simulink model "VSI"  (Simulink 8.2)
settings: Solver=ode23t  StartTime=0  StopTime=0.01  MaxStep=.1e-6  RelTol=1e-4  AbsTol=1e-5
values from neighbouring files (symbols this model uses):
  Ca = 1/1*32e-6    (= 3.2e-05)    [VSI_AFE_parameters_LC_900Hz.m]    (also in VSI_AFE_parameters_LC_9kHz.m = 1.6e-05)
  Cc = 1/1*31.8e-6    (= 3.18e-05)    [VSI_AFE_parameters_LC_900Hz.m]    (also in VSI_AFE_parameters_LC_9kHz.m = 1.59e-05)
  Cdc_vsi = 147.3e-6    (= 0.0001473)    [VSI_AFE_parameters_LC_900Hz.m]    (also in VSI_AFE_parameters_LC_9kHz.m)
  DeadTime = 0*0.5e-6    (= 0)    [VSI_AFE_parameters_LC_900Hz.m]    (also in VSI_AFE_parameters_LC_9kHz.m)
  FWPI_a1 = 0.08921    [VSI_AFE_parameters_LC_900Hz.m]    (also in VSI_AFE_parameters_LC_9kHz.m)
  FWPI_a2 = -0.08901    [VSI_AFE_parameters_LC_900Hz.m]    (also in VSI_AFE_parameters_LC_9kHz.m)
  Kii_AFE = 46.5421*270    (= 12566.367)    [VSI_AFE_parameters_LC_900Hz.m]    (also in VSI_AFE_parameters_LC_9kHz.m)
  Kii_VSI = 121.0095*270    (= 32672.565)    [VSI_AFE_parameters_LC_900Hz.m]    (also in VSI_AFE_parameters_LC_9kHz.m)
  Kiv_AFE = 4.5815    [VSI_AFE_parameters_LC_900Hz.m]    (also in VSI_AFE_parameters_LC_9kHz.m)
  Kiv_VSI = 130.8997    [VSI_AFE_parameters_LC_900Hz.m]    (also in VSI_AFE_parameters_LC_9kHz.m)
  Kpi_AFE = 0.0116*270    (= 3.132)    [VSI_AFE_parameters_LC_900Hz.m]    (also in VSI_AFE_parameters_LC_9kHz.m)
  Kpi_VSI = 0.0465*270    (= 12.555)    [VSI_AFE_parameters_LC_900Hz.m]    (also in VSI_AFE_parameters_LC_9kHz.m)
  Kpv_AFE = 0.0462    [VSI_AFE_parameters_LC_900Hz.m]    (also in VSI_AFE_parameters_LC_9kHz.m)
  Kpv_VSI = 0.0495    [VSI_AFE_parameters_LC_900Hz.m]    (also in VSI_AFE_parameters_LC_9kHz.m)
  La = 1/1*962e-6    (= 0.000962)    [VSI_AFE_parameters_LC_900Hz.m]    (also in VSI_AFE_parameters_LC_9kHz.m = 1.924e-05)
  Lb = 1/1*985e-6    (= 0.000985)    [VSI_AFE_parameters_LC_900Hz.m]    (also in VSI_AFE_parameters_LC_9kHz.m = 1.97e-05)
  Lc = 1/1*972e-6    (= 0.000972)    [VSI_AFE_parameters_LC_900Hz.m]    (also in VSI_AFE_parameters_LC_9kHz.m = 1.944e-05)
  LCa = 0.61e-6    (= 6.1e-07)    [VSI_AFE_parameters_LC_900Hz.m]    (also in VSI_AFE_parameters_LC_9kHz.m)
  LCb = 0.61e-6    (= 6.1e-07)    [VSI_AFE_parameters_LC_900Hz.m]    (also in VSI_AFE_parameters_LC_9kHz.m)
  LCc = 0.63e-6    (= 6.3e-07)    [VSI_AFE_parameters_LC_900Hz.m]    (also in VSI_AFE_parameters_LC_9kHz.m)
  LCdc_vsi = 0.57e-6    (= 5.7e-07)    [VSI_AFE_parameters_LC_900Hz.m]    (also in VSI_AFE_parameters_LC_9kHz.m)
  PWM_Cycle = 4000    [VSI_AFE_parameters_LC_900Hz.m]    (also in VSI_AFE_parameters_LC_9kHz.m)
  R = 12    [VSI_AFE_parameters_LC_900Hz.m]    (also in VSI_AFE_parameters_LC_9kHz.m)
  RCa = 0.051    [VSI_AFE_parameters_LC_900Hz.m]    (also in VSI_AFE_parameters_LC_9kHz.m)
  RCb = 0.054    [VSI_AFE_parameters_LC_900Hz.m]    (also in VSI_AFE_parameters_LC_9kHz.m)
  RCc = 0.052    [VSI_AFE_parameters_LC_900Hz.m]    (also in VSI_AFE_parameters_LC_9kHz.m)
  RCdc_vsi = 0.046    [VSI_AFE_parameters_LC_900Hz.m]    (also in VSI_AFE_parameters_LC_9kHz.m)
  RLa = 0.123    [VSI_AFE_parameters_LC_900Hz.m]    (also in VSI_AFE_parameters_LC_9kHz.m)
  RLb = 0.132    [VSI_AFE_parameters_LC_900Hz.m]    (also in VSI_AFE_parameters_LC_9kHz.m)
  RLc = 0.089    [VSI_AFE_parameters_LC_900Hz.m]    (also in VSI_AFE_parameters_LC_9kHz.m)
  Vdc = 270/1    (= 270)    [VSI_AFE_parameters_LC_900Hz.m]    (also in VSI_AFE_parameters_LC_9kHz.m)
undefined symbols (not defined in the file or in its folder): Cdc, Ldc
libraries: powerlib x27, cstblocks x10, powerlib_extras x3, simulink x2
settings Model: Creator=marko  LastModifiedBy=wenbo
settings SolverCC: MaxConsecutiveMinStep=10  ZeroCrossAlgorithm=Adaptive  AlgebraicLoopSolver=LineSearch
settings DataIOCC: LimitDataPoints=off  SaveFinalState=on
settings DebuggingCC: IgnoredZcDiagnostic=none  FcnCallInpInsideContextMsg=EnableAllAsWarning

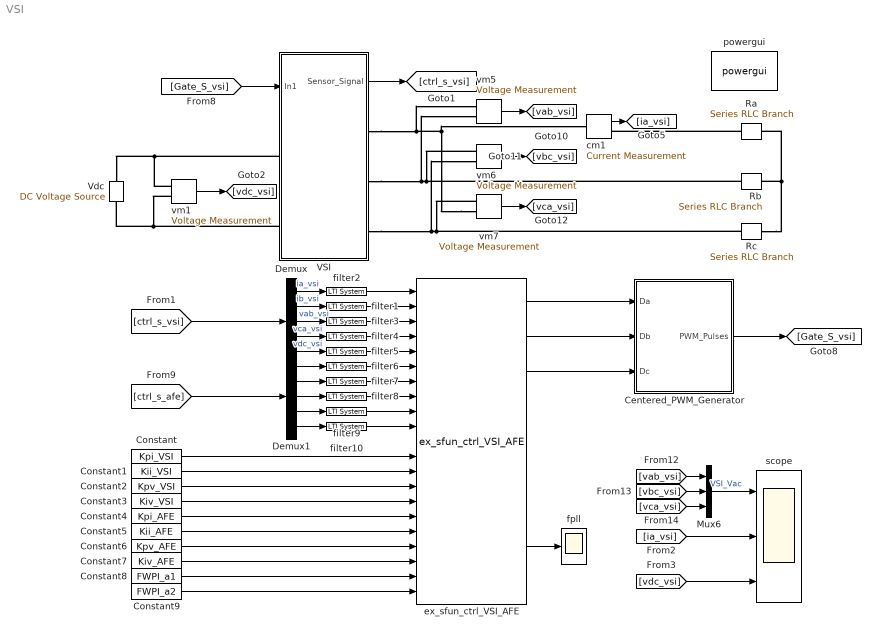
== system VSI ==
  Centered_PWM_Generator : Subsystem
  Constant : Constant  Value=Kpi_VSI
  Constant1 : Constant  Value=Kii_VSI
  Constant2 : Constant  Value=Kpv_VSI
  Constant3 : Constant  Value=Kiv_VSI
  Constant4 : Constant  Value=Kpi_AFE
  Constant5 : Constant  Value=Kii_AFE
  Constant6 : Constant  Value=Kpv_AFE
  Constant7 : Constant  Value=Kiv_AFE
  Constant8 : Constant  Value=FWPI_a1
  Constant9 : Constant  Value=FWPI_a2
  Demux : Demux  Outputs=5
  Demux1 : Demux  Outputs=5
  Mux6 : Mux  Inputs=3
  Ra : powerlib/Elements/Series RLC Branch  LConnTagsString=__new0  RConnTagsString=__new0  BranchType=R  Resistance=R  Inductance=Ldc  SetiL0=off  InitialCurrent=0  Capacitance=Cdc  Setx0=off  InitialVoltage=0  Measurements=None
  Rb : powerlib/Elements/Series RLC Branch  LConnTagsString=__new0  RConnTagsString=__new0  BranchType=R  Resistance=R  Inductance=Ldc  SetiL0=off  InitialCurrent=0  Capacitance=Cdc  Setx0=off  InitialVoltage=0  Measurements=None
  Rc : powerlib/Elements/Series RLC Branch  LConnTagsString=__new0  RConnTagsString=__new0  BranchType=R  Resistance=R  Inductance=Ldc  SetiL0=off  InitialCurrent=0  Capacitance=Cdc  Setx0=off  InitialVoltage=0  Measurements=None
  VSI : Subsystem
  Vdc : powerlib/Electrical Sources/DC Voltage Source  Amplitude=Vdc  Measurements=None
  cm1 : powerlib/Measurements/Current Measurement  PhasorSimulation=off  OutputType=Complex  PSBequivalent=0
  ex_sfun_ctrl_VSI_AFE : S-Function  FunctionName=ex_sfun_ctrl_VSI_AFE  EnableBusSupport=off
  filter{1..10} (10 alike) : cstblocks/LTI System  sys=tf_filter  IC=[]
  fpll : Scope
      settings: TimeRange=0.4  YMin=-150  YMax=60  SaveName=ia_L1
  powergui : powerlib/powergui  Priority=1  SimulationMode=Continuous  SolverType=Tustin  SampleTime=50e-6  frequency=60  SPID=on  DisableSnubberDevices=off  DisableRonSwitches=off  DisableVfSwitches=off  SwTol=0  Interpol=off  DisplayEquations=off  frequencyindice=0  Pbase=100e6  ErrMax=1e-4  Iterations=50  UnitsV=kV  UnitsW=MW  FunctionMessages=off  echomessages=off  HookPort=off  EnableUseOfTLC=off  x0status=blocks  RestoreLinks=warning  ResistiveCurrentMeasurement=off  Frange=[0:2:500]  Ylog=off  Xlog=on  ShowGrid=off  save=off  variable=ZData  structure=ia_L  ZoomFFT=on  StartTime=0.1  cycles=1  DisplayStyle=1  fundamental=400  FreqAxis=off  MaxFrequency=100000  frequencyindicesteady=400  RmsSteady=1  display=off  Ts=0  methode=off
  scope : Scope  NumInputPorts=3
      settings: YMin=-150~-8~-1  YMax=150~8~1  SaveName=va_ia  MaxDataPoints=2000000
  vm{1,5..7} (4 alike) : powerlib/Measurements/Voltage Measurement  PhasorSimulation=off  OutputType=Complex  PSBequivalent=0
  wires:
  vm5/1 -> [vab_vsi]
  vm6/1 -> [vbc_vsi]
  vm7/1 -> [vca_vsi]
  [vab_vsi] -> Mux6/1
  [vbc_vsi] -> Mux6/2
  [vca_vsi] -> Mux6/3
  Mux6/1 -> scope/1  "VSI_Vac"
  Centered_PWM_Generator/1(PWM_Pulses) -> [Gate_S_vsi]
  VSI/1(Sensor_Signal) -> [ctrl_s_vsi]
  [Gate_S_vsi] -> VSI/1(In1)
  [ctrl_s_afe] -> Demux1/1
  ex_sfun_ctrl_VSI_AFE/1 -> Centered_PWM_Generator/1(Da)
  ex_sfun_ctrl_VSI_AFE/2 -> Centered_PWM_Generator/2(Db)
  ex_sfun_ctrl_VSI_AFE/3 -> Centered_PWM_Generator/3(Dc)
  ex_sfun_ctrl_VSI_AFE/8 -> fpll/1
  cm1/1 -> [ia_vsi]
  [ia_vsi] -> scope/2
  [vdc_vsi] -> scope/3
  [ctrl_s_vsi] -> Demux/1
  Demux/1 -> filter2/1  "ia_vsi"
  Demux/2 -> filter1/1  "ib_vsi"
  Demux/3 -> filter3/1  "vab_vsi"
  Demux/4 -> filter4/1  "vca_vsi"
  Demux/5 -> filter5/1  "vdc_vsi"
  Demux1/1 -> filter6/1
  Demux1/2 -> filter7/1
  Demux1/3 -> filter8/1
  Demux1/4 -> filter9/1
  Demux1/5 -> filter10/1
  Constant/1 -> ex_sfun_ctrl_VSI_AFE/12
  Constant1/1 -> ex_sfun_ctrl_VSI_AFE/13
  Constant2/1 -> ex_sfun_ctrl_VSI_AFE/14
  Constant3/1 -> ex_sfun_ctrl_VSI_AFE/15
  Constant4/1 -> ex_sfun_ctrl_VSI_AFE/16
  Constant5/1 -> ex_sfun_ctrl_VSI_AFE/17
  Constant6/1 -> ex_sfun_ctrl_VSI_AFE/18
  Constant7/1 -> ex_sfun_ctrl_VSI_AFE/19
  Constant8/1 -> ex_sfun_ctrl_VSI_AFE/20
  Constant9/1 -> ex_sfun_ctrl_VSI_AFE/21
  filter2/1 -> ex_sfun_ctrl_VSI_AFE/1
  filter1/1 -> ex_sfun_ctrl_VSI_AFE/2
  filter3/1 -> ex_sfun_ctrl_VSI_AFE/3
  filter4/1 -> ex_sfun_ctrl_VSI_AFE/4
  filter5/1 -> ex_sfun_ctrl_VSI_AFE/5
  filter6/1 -> ex_sfun_ctrl_VSI_AFE/6
  filter7/1 -> ex_sfun_ctrl_VSI_AFE/7
  filter8/1 -> ex_sfun_ctrl_VSI_AFE/8
  filter9/1 -> ex_sfun_ctrl_VSI_AFE/9
  filter10/1 -> ex_sfun_ctrl_VSI_AFE/10
  vm1/1 -> [vdc_vsi]
  connections:
  VSI/LConn1 -- vm1/LConn1 -- Vdc/RConn1
  VSI/LConn2 -- vm1/LConn2 -- Vdc/LConn1
  vm7/LConn1 -- VSI/RConn3 -- vm6/LConn2 -- Rc/RConn1
  vm6/LConn1 -- VSI/RConn2 -- vm5/LConn2 -- Rb/RConn1
  Rb/LConn1 -- Rc/LConn1 -- Ra/LConn1
  vm7/LConn2 -- VSI/RConn1 -- vm5/LConn1 -- cm1/LConn1
  Ra/RConn1 -- cm1/RConn1

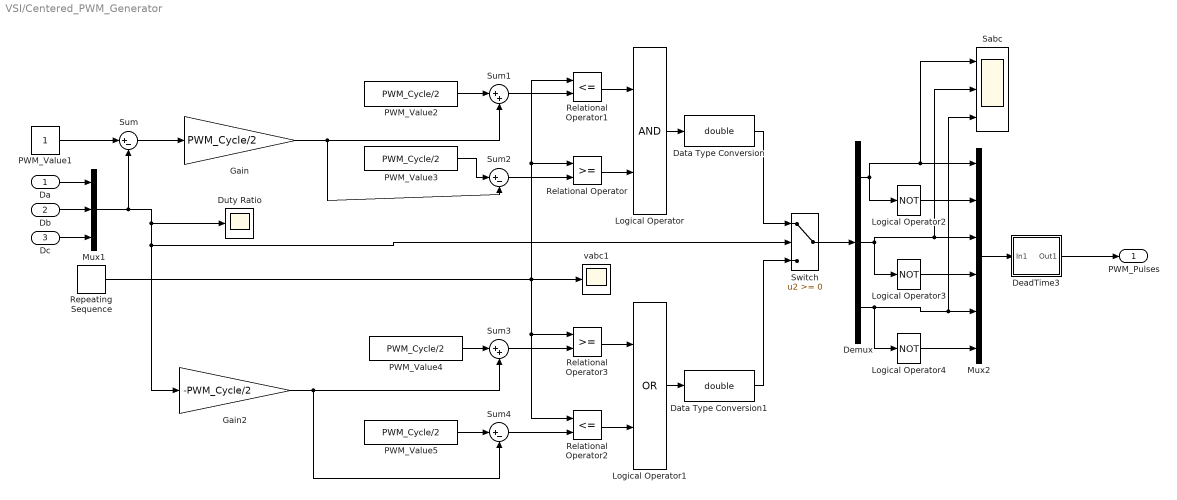
== system VSI/Centered_PWM_Generator ==
  Da : Inport
  Db : Inport  Port=2
  Dc : Inport  Port=3
  Data Type Conversion : DataTypeConversion  OutDataTypeStr=double
  Data Type Conversion1 : DataTypeConversion  OutDataTypeStr=double
  DeadTime3 : Subsystem
  Demux : Demux  Outputs=3
  Duty Ratio : Scope
      settings: TimeRange=0.01  YMin=0.25  YMax=0.75  SaveName=vabcll1
  Gain : Gain  Gain=PWM_Cycle/2
  Gain2 : Gain  Gain=-PWM_Cycle/2
  Logical Operator : Logic  AllPortsSameDT=off  OutDataTypeStr=boolean
  Logical Operator1 : Logic  Operator=OR  AllPortsSameDT=off  OutDataTypeStr=boolean
  Logical Operator2 : Logic  Operator=NOT  OutDataTypeStr=float('double')
  Logical Operator3 : Logic  Operator=NOT  OutDataTypeStr=float('double')
  Logical Operator4 : Logic  Operator=NOT  OutDataTypeStr=float('double')
  Mux1 : Mux  Inputs=3
  Mux2 : Mux  Inputs=6
  PWM_Value1 : Constant
  PWM_Value{2..5} (4 alike) : Constant  Value=PWM_Cycle/2
  Relational Operator : RelationalOperator  OutDataTypeStr=boolean
  Relational Operator1 : RelationalOperator  Operator=<=  OutDataTypeStr=boolean
  Relational Operator2 : RelationalOperator  Operator=<=  OutDataTypeStr=boolean
  Relational Operator3 : RelationalOperator  OutDataTypeStr=boolean
  Repeating Sequence : simulink/Sources/Repeating Sequence  rep_seq_t="[0  (PWM_Cycle*12.5e-9)]"  rep_seq_y=[0 PWM_Cycle]
  Sabc : Scope  NumInputPorts=3
      settings: TimeRange=0.0005  YMin=-9~-5~-5  YMax=8~5~5  SaveName=iabc_L2
  Sum : Sum  Inputs=|+-
  Sum1 : Sum  Inputs=|++
  Sum2 : Sum  Inputs=|+-
  Sum3 : Sum  Inputs=|++
  Sum4 : Sum  Inputs=|+-
  Switch : Switch
  vabc1 : Scope
      settings: TimeRange=0.01  YMin=0  YMax=4000  SaveName=vabcll2
  PWM_Pulses : Outport
  wires:
  Logical Operator4/1 -> Mux2/6
  Demux/3 -> Logical Operator4/1, Mux2/5, Sabc/3
  Logical Operator3/1 -> Mux2/4
  Demux/2 -> Mux2/3, Sabc/2, Logical Operator3/1
  Logical Operator2/1 -> Mux2/2
  Demux/1 -> Mux2/1, Sabc/1, Logical Operator2/1
  Mux2/1 -> DeadTime3/1(In1)
  Dc/1 -> Mux1/3
  Db/1 -> Mux1/2
  Da/1 -> Mux1/1
  Mux1/1 -> Sum/2, Gain2/1, Switch/2, Duty Ratio/1
  Switch/1 -> Demux/1
  Data Type Conversion1/1 -> Switch/3
  Gain2/1 -> Sum3/2, Sum4/2
  Logical Operator1/1 -> Data Type Conversion1/1
  Relational Operator2/1 -> Logical Operator1/2
  Relational Operator3/1 -> Logical Operator1/1
  Sum3/1 -> Relational Operator3/2
  Sum4/1 -> Relational Operator2/2
  PWM_Value5/1 -> Sum4/1
  PWM_Value4/1 -> Sum3/1
  Data Type Conversion/1 -> Switch/1
  Logical Operator/1 -> Data Type Conversion/1
  Relational Operator/1 -> Logical Operator/2
  Relational Operator1/1 -> Logical Operator/1
  Sum1/1 -> Relational Operator1/2
  Sum2/1 -> Relational Operator/2
  PWM_Value3/1 -> Sum2/1
  Gain/1 -> Sum2/2, Sum1/2
  Sum/1 -> Gain/1
  PWM_Value1/1 -> Sum/1
  Repeating Sequence/1 -> vabc1/1, Relational Operator1/1, Relational Operator/1, Relational Operator3/1, Relational Operator2/1
  DeadTime3/1(Out1) -> PWM_Pulses/1
  PWM_Value2/1 -> Sum1/1

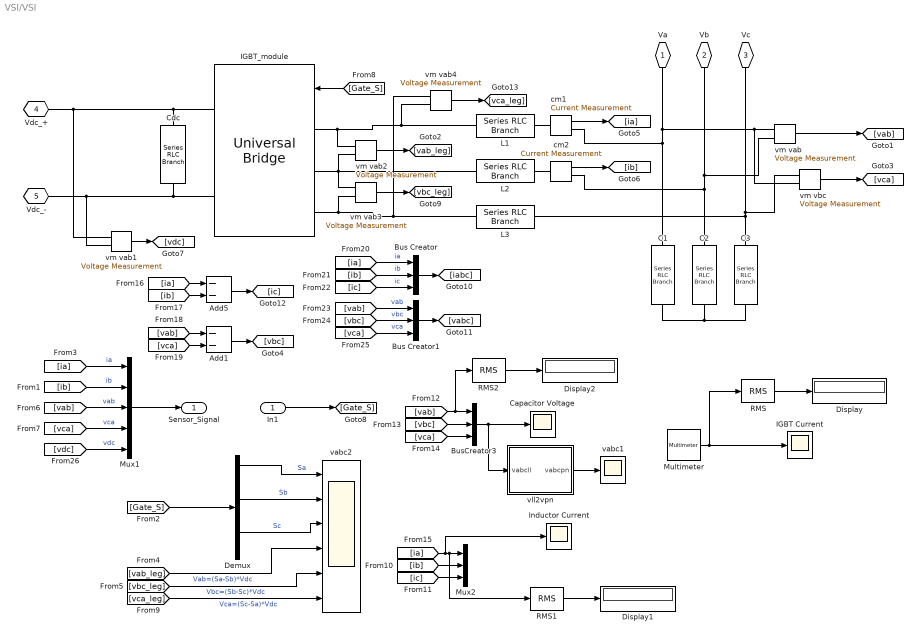
== system VSI/VSI ==
  In1 : Inport
  Add1 : Sum  Inputs=--
  Add5 : Sum  Inputs=--
  Bus Creator : BusCreator  Inputs=3
  Bus Creator1 : BusCreator  Inputs=3
  BusCreator3 : BusCreator  Inputs=3
  C1 : powerlib/Elements/Series RLC Branch  LConnTagsString=__new0  RConnTagsString=__new0  BranchType=RC  Resistance=RCa  Inductance=LCa  SetiL0=off  InitialCurrent=0  Capacitance=Ca  Setx0=off  InitialVoltage=0  Measurements=None
  C2 : powerlib/Elements/Series RLC Branch  LConnTagsString=__new0  RConnTagsString=__new0  BranchType=RC  Resistance=RCb  Inductance=LCb  SetiL0=off  InitialCurrent=0  Capacitance=Cc  Setx0=off  InitialVoltage=0  Measurements=None
  C3 : powerlib/Elements/Series RLC Branch  LConnTagsString=__new0  RConnTagsString=__new0  BranchType=RC  Resistance=RCc  Inductance=LCc  SetiL0=off  InitialCurrent=0  Capacitance=Cc  Setx0=off  InitialVoltage=0  Measurements=None
  Capacitor Voltage : Scope
      settings: TimeRange=0.06  YMin=-300  YMax=225  SaveName=vabcll
  Cdc : powerlib/Elements/Series RLC Branch  LConnTagsString=__new0  RConnTagsString=__new0  BranchType=RC  Resistance=RCdc_vsi  Inductance=LCdc_vsi  SetiL0=off  InitialCurrent=0  Capacitance=Cdc_vsi  Setx0=off  InitialVoltage=0  Measurements=None
  Demux : Demux  Outputs=6
  Display : Display
  Display1 : Display
  Display2 : Display
  IGBT Current : Scope
      settings: TimeRange=0.01  YMin=-80  YMax=80  SaveName=I_IGBT
  IGBT_module : powerlib/Power Electronics/Universal Bridge  Arms=3  SnubberResistance=inf  SnubberCapacitance=inf  Device=IGBT / Diodes  Ron=0  Lon=0  ForwardVoltages=[0 0]  ForwardVoltage=0  GTOparameters=[ 10e-6 , 20e-6 ]  IGBTparameters=[ 0, 0 ]  Measurements=All voltages and currents  Measurements_2=None  converterType=Rectifier
  Inductor Current : Scope
      settings: TimeRange=0.06  YMin=-35  YMax=35  SaveName=Ia_L
  L1 : powerlib/Elements/Series RLC Branch  LConnTagsString=__new0  RConnTagsString=__new0  BranchType=RL  Resistance=RLa  Inductance=La  SetiL0=off  InitialCurrent=0  Capacitance=1e-6  Setx0=off  InitialVoltage=0  Measurements=None
  L2 : powerlib/Elements/Series RLC Branch  LConnTagsString=__new0  RConnTagsString=__new0  BranchType=RL  Resistance=RLb  Inductance=Lb  SetiL0=off  InitialCurrent=0  Capacitance=1e-6  Setx0=off  InitialVoltage=0  Measurements=None
  L3 : powerlib/Elements/Series RLC Branch  LConnTagsString=__new0  RConnTagsString=__new0  BranchType=RL  Resistance=RLc  Inductance=Lc  SetiL0=off  InitialCurrent=0  Capacitance=1e-6  Setx0=off  InitialVoltage=0  Measurements=None
  Multimeter : powerlib/Measurements/Multimeter  PhasorSimulation=off  OutputType=Complex  sel=11  L=16  Gain=1  yselected={'Isw1: VSI/IGBT_module'};  PSBOutputType=1  PSBequivalent=0  AxesSetting=[0,0.1,-100,100]  Display=0  SavedBlockNames=-11
  Mux1 : Mux  Inputs=5
  Mux2 : Mux  Inputs=3
  RMS : powerlib_extras/Measurements/RMS  f1=400
  RMS1 : powerlib_extras/Measurements/RMS  f1=400
  RMS2 : powerlib_extras/Measurements/RMS  f1=400
  cm1 : powerlib/Measurements/Current Measurement  PhasorSimulation=off  OutputType=Complex  PSBequivalent=0
  cm2 : powerlib/Measurements/Current Measurement  PhasorSimulation=off  OutputType=Complex  PSBequivalent=0
  vabc1 : Scope
      settings: TimeRange=0.01  YMin=-80  YMax=80  SaveName=vabc
  vabc2 : Scope  NumInputPorts=6
      settings: YMin=0~0~0~-300~-300~-300  YMax=1~1~1~300~300~300  SaveName=gate_vab
  vll2vpn : Subsystem
  vm vab{,1..4} (5 alike) : powerlib/Measurements/Voltage Measurement  PhasorSimulation=off  OutputType=Complex  PSBequivalent=0
  vm vbc : powerlib/Measurements/Voltage Measurement  PhasorSimulation=off  OutputType=Complex  PSBequivalent=0
  Va : PMIOPort  Tag=PMCPort  Port=1  Side=Right
  Vb : PMIOPort  Tag=PMCPort  Port=2  Side=Right
  Vc : PMIOPort  Tag=PMCPort  Port=3  Side=Right
  Vdc_+ : PMIOPort  Tag=PMCPort  Port=4  Side=Left
  Vdc_- : PMIOPort  Tag=PMCPort  Port=5  Side=Left
  Sensor_Signal : Outport
  wires:
  cm1/1 -> [ia]
  [Gate_S] -> IGBT_module/1
  BusCreator3/1 -> Capacitor Voltage/1, vll2vpn/1(vabcll)
  [vab] -> RMS2/1, BusCreator3/1
  [vbc] -> BusCreator3/2
  [vca] -> BusCreator3/3
  [ia] -> Bus Creator/1  "ia"
  [ib] -> Bus Creator/2  "ib"
  [ic] -> Bus Creator/3  "ic"
  Bus Creator/1 -> [iabc]
  [vab] -> Bus Creator1/1  "vab"
  [vbc] -> Bus Creator1/2  "vbc"
  [vca] -> Bus Creator1/3  "vca"
  Bus Creator1/1 -> [vabc]
  vll2vpn/1(vabcpn) -> vabc1/1
  RMS/1 -> Display/1
  cm2/1 -> [ib]
  vm vab/1 -> [vab]
  vm vbc/1 -> [vca]
  vm vab1/1 -> [vdc]
  [ia] -> Mux1/1  "ia"
  [ib] -> Mux1/2  "ib"
  [vab] -> Mux1/3  "vab"
  [vca] -> Mux1/4  "vca"
  [vdc] -> Mux1/5  "vdc"
  Mux1/1 -> Sensor_Signal/1
  In1/1 -> [Gate_S]
  Add5/1 -> [ic]
  [ia] -> Add5/1
  [ib] -> Add5/2
  Add1/1 -> [vbc]
  [vab] -> Add1/1
  [vca] -> Add1/2
  RMS1/1 -> Display1/1
  Demux/1 -> vabc2/1  "Sa"
  Demux/3 -> vabc2/2  "Sb"
  Demux/5 -> vabc2/3  "Sc"
  [Gate_S] -> Demux/1
  vm vab2/1 -> [vab_leg]
  vm vab3/1 -> [vbc_leg]
  vm vab4/1 -> [vca_leg]
  [vab_leg] -> vabc2/4  "Vab=(Sa-Sb)*Vdc"
  [vbc_leg] -> vabc2/5  "Vbc=(Sb-Sc)*Vdc"
  [vca_leg] -> vabc2/6  "Vca=(Sc-Sa)*Vdc"
  Multimeter/1 -> IGBT Current/1, RMS/1
  RMS2/1 -> Display2/1
  [ib] -> Mux2/2
  [ic] -> Mux2/3
  [ia] -> Inductor Current/1, RMS1/1, Mux2/1
  connections:
  Va/RConn1 -- cm1/RConn1 -- C1/LConn1 -- vm vab/LConn1 -- vm vbc/LConn2
  C3/RConn1 -- C2/RConn1 -- C1/RConn1
  vm vab/LConn2 -- cm2/RConn1 -- C2/LConn1 -- Vb/RConn1
  L1/LConn1 -- vm vab4/LConn2 -- vm vab2/LConn1 -- IGBT_module/LConn1
  L1/RConn1 -- cm1/LConn1
  L2/RConn1 -- cm2/LConn1
  IGBT_module/LConn2 -- vm vab3/LConn1 -- vm vab2/LConn2 -- L2/LConn1
  L3/LConn1 -- vm vab4/LConn1 -- vm vab3/LConn2 -- IGBT_module/LConn3
  Vdc_+/RConn1 -- IGBT_module/RConn1 -- Cdc/LConn1 -- vm vab1/LConn1
  Vdc_-/RConn1 -- IGBT_module/RConn2 -- Cdc/RConn1 -- vm vab1/LConn2
  Vc/RConn1 -- C3/LConn1 -- L3/RConn1 -- vm vbc/LConn1

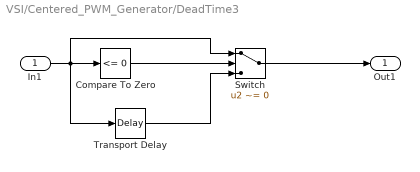
== system VSI/Centered_PWM_Generator/DeadTime3 ==
  In1 : Inport
  Compare To Zero : simulink/Logic and Bit Operations/Compare To Zero  relop=<=  OutDataTypeStr=uint8
  Switch : Switch  Criteria=u2 ~= 0
  Transport Delay : TransportDelay  DelayTime=DeadTime  BufferSize=2048*16  FixedBuffer=on
  Out1 : Outport
  wires:
  Switch/1 -> Out1/1
  Compare To Zero/1 -> Switch/2
  Transport Delay/1 -> Switch/3
  In1/1 -> Transport Delay/1, Compare To Zero/1, Switch/1

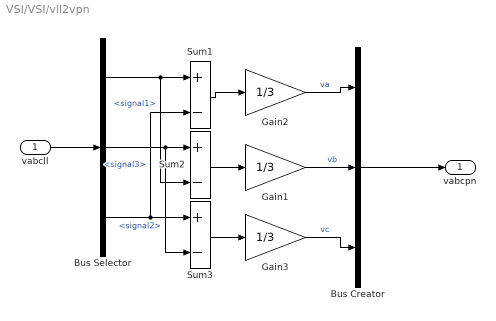
== system VSI/VSI/vll2vpn ==
  vabcll : Inport
  Bus Creator : BusCreator  Inputs=3
  Bus Selector : BusSelector
  Gain1 : Gain  Gain=1/3
  Gain2 : Gain  Gain=1/3
  Gain3 : Gain  Gain=1/3
  Sum1 : Sum  Inputs=+-
  Sum2 : Sum  Inputs=+-
  Sum3 : Sum  Inputs=+-
  vabcpn : Outport
  wires:
  Bus Creator/1 -> vabcpn/1
  vabcll/1 -> Bus Selector/1
  Bus Selector/1 -> Sum1/1, Sum2/2  "<signal1>"
  Bus Selector/3 -> Sum1/2, Sum3/1  "<signal3>"
  Sum1/1 -> Gain2/1
  Bus Selector/2 -> Sum2/1, Sum3/2  "<signal2>"
  Sum2/1 -> Gain1/1
  Sum3/1 -> Gain3/1
  Gain2/1 -> Bus Creator/1  "va"
  Gain1/1 -> Bus Creator/2  "vb"
  Gain3/1 -> Bus Creator/3  "vc"
